simulink model "RLC_with_HBrdige_forward_circuit"  (R2022a)
settings: Solver=FixedStepAuto  StartTime=0.0  StopTime=.004  FixedStep=1e-6  RelTol=1e-3
values from neighbouring files (symbols this model uses):
  amplitude = 1200/pi    (= 381.971863421)    [RLC_Square_Wave_Driver.m]
  period = loc_nada(3) - loc_nada(1)    [Phase_shifting.m]    (also in RLC_Square_Wave_Driver.m = 1/i)
  RunTime = .004    (= 0.004)    [All_injectors_LQG_bop_plasma_ss_model_code.m]    (also in All_injectors_LQG_bop_ss_model_code.m; All_injectors_LQG_continuous_time_code.m; All_injectors_LQG_plasma_7_15_24_code.m; All_injectors_LQG_plasma_ss_model_code.m)
libraries: spsSeriesRLCBranchLib x8, spsMosfetLib x4, spsVoltageMeasurementLib x4, spsDCVoltageSourceLib x3, spsFullBridgeMMCExternalDCLinksLib x2, spsOnDelayLib x2, spsPWMGeneratorMultilevelLib x2, spsCurrentMeasurementLib x2, simulink x1, spspowerguiLib x1
settings Model: Creator=ducks  LastModifiedBy=ducks
settings DataIOCC: ExternalInput=[t,V]

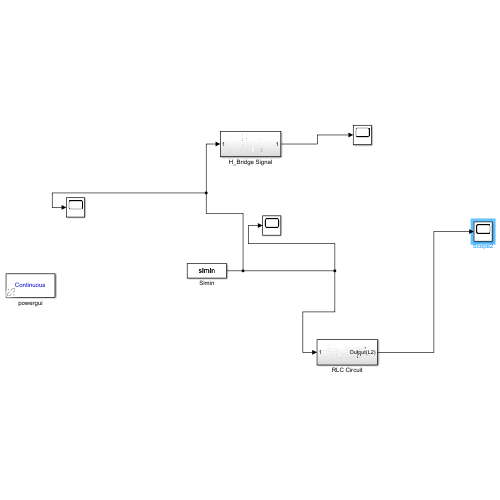
[thumbnail: Simulink's stored preview of the top-level diagram]
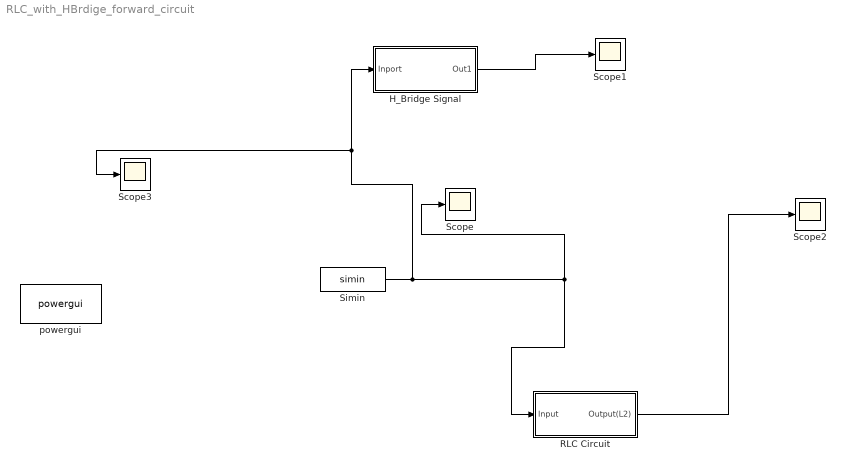
== system RLC_with_HBrdige_forward_circuit ==
  H_Bridge Signal : Subsystem
  RLC Circuit : Subsystem
  Scope{,1..3} (4 alike) : Scope
  Simin : FromWorkspace  VariableName=simin
  powergui : spspowerguiLib/powergui  Priority=1  SimulationMode=Continuous  SampleTime=50e-6  frequency=60  Iterations=50  frequencyindice=0  Pbase=100e6  ErrMax=1e-4  UnitsV=kV  UnitsW=MW  buscounter=0  FunctionMessages=off  echomessages=off  EnableUseOfTLC=off  CurrentSourceSwitches=off  DisableSnubberDevices=off  DisableRonSwitches=off  DisableVfSwitches=off  DisplayEquations=off  AutomaticDiscreteSolvers=off  SolverType=Tustin/Backward Euler (TBE)  Interpol=off  ExternalGateDelay=off  methode=off  Ts=100  x0status=blocks  SPID=on  SwTol=0  HookPort=off  NonlinearTolerance=1e-4  nMaxIteration=100  ContinueOnMaxIteration=off  RestoreLinks=warning  ResistiveCurrentMeasurement=off  Frange=[0:2:500]  Ylog=off  Xlog=on  ShowGrid=off  save=off  variable=ZData  structure=0  ZoomFFT=off  StartTime=0.0  cycles=1  DisplayStyle=1  fundamental=60  FreqAxis=off  MaxFrequency=1000  frequencyindicesteady=1  RmsSteady=1  display=off
  wires:
  Simin/1 -> Scope3/1, H_Bridge Signal/1(Inport), Scope/1, RLC Circuit/1(Input)
  H_Bridge Signal/1(Out1) -> Scope1/1
  RLC Circuit/1(Output(L2)) -> Scope2/1

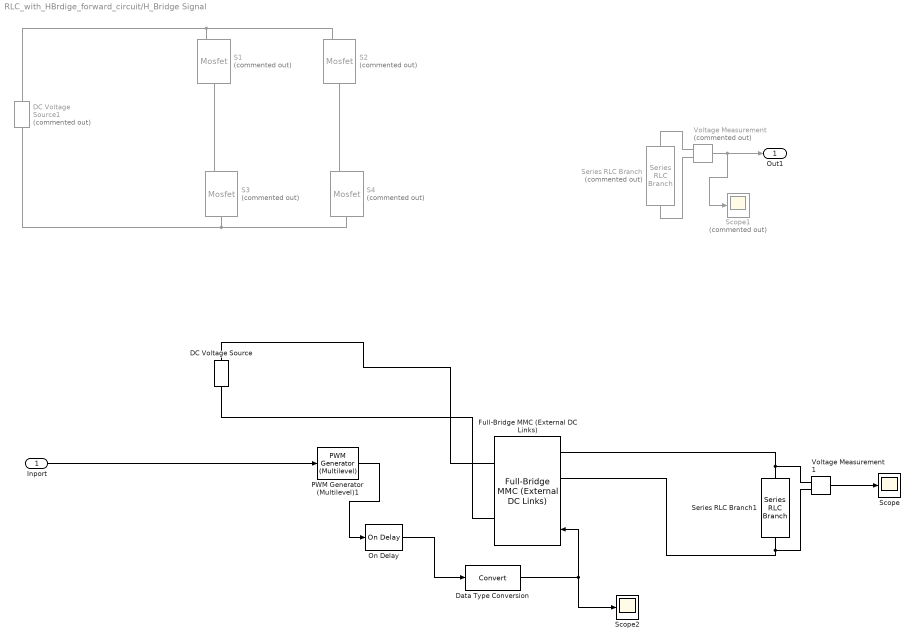
== system RLC_with_HBrdige_forward_circuit/H_Bridge Signal ==
  Inport : Inport
  DC Voltage Source : spsDCVoltageSourceLib/DC Voltage Source  Amplitude=600  Measurements=None
  DC Voltage Source1 : spsDCVoltageSourceLib/DC Voltage Source  Commented=on  Amplitude=600  Measurements=None
  Data Type Conversion : DataTypeConversion  SaturateOnIntegerOverflow=off  RndMeth=Floor
  Full-Bridge MMC (External DC Links) : spsFullBridgeMMCExternalDCLinksLib/Full-Bridge MMC (External DC Links)  ModelType=Switching devices  n=1  Ron=1e-3  Rs=1e6  Cs=inf  Ron_Diode=1e-3  Rs_Diode=1e6  Cs_Diode=inf  Vf_Diode=1e-3  Rs_CurrentSource=inf  Ts=10e-6
      settings: SourceProductBaseCode=PS
  On Delay : spsOnDelayLib/On Delay  DelayType=On delay  delay=.05*period  ic=0  Ts=0
      settings: SourceProductBaseCode=PS
  PWM Generator (Multilevel)1 : spsPWMGeneratorMultilevelLib/PWM Generator (Multilevel)  BridgeType=Full-bridge  NumberOfBridges=1  Fc=1e3  Ts=0  ShowCarriersOutport=off
      settings: SourceProductBaseCode=PS
  S{1..4} (4 alike) : spsMosfetLib/Mosfet  Commented=on  Ron=0.1  Lon=0  Rd=0.01  Vfd=0  IC=0  Rs=1e5  Cs=inf  Measurements=off
  Scope : Scope
  Scope1 : Scope  Commented=on
  Scope2 : Scope
  Series RLC Branch : spsSeriesRLCBranchLib/Series RLC Branch  Commented=on  LConnTagsString=__new0  RConnTagsString=__new0  BranchType=R  Resistance=1  Inductance=1e-3  SetiL0=off  InitialCurrent=0  Capacitance=1e-6  Setx0=off  InitialVoltage=0  Measurements=None
  Series RLC Branch1 : spsSeriesRLCBranchLib/Series RLC Branch  LConnTagsString=__new0  RConnTagsString=__new0  BranchType=R  Resistance=1  Inductance=1e-3  SetiL0=off  InitialCurrent=0  Capacitance=1e-6  Setx0=off  InitialVoltage=0  Measurements=None
  Voltage Measurement : spsVoltageMeasurementLib/Voltage Measurement  Commented=on  PhasorSimulation=off  OutputType=Complex  PSBequivalent=0
  Voltage Measurement1 : spsVoltageMeasurementLib/Voltage Measurement  PhasorSimulation=off  OutputType=Complex  PSBequivalent=0
  Out1 : Outport
  wires:
  Voltage Measurement/1 -> Scope1/1, Out1/1
  On Delay/1 -> Data Type Conversion/1
  PWM Generator (Multilevel)1/1 -> On Delay/1
  Inport/1 -> PWM Generator (Multilevel)1/1
  Data Type Conversion/1 -> Full-Bridge MMC (External DC Links)/1, Scope2/1
  Voltage Measurement1/1 -> Scope/1
  connections:
  Voltage Measurement/LConn1 -- Series RLC Branch/LConn1
  Voltage Measurement/LConn2 -- Series RLC Branch/RConn1
  S1/LConn1 -- S2/LConn1 -- DC Voltage Source1/LConn1
  S1/RConn1 -- S3/LConn1
  S3/RConn1 -- DC Voltage Source1/RConn1 -- S4/RConn1
  S4/LConn1 -- S2/RConn1
  Full-Bridge MMC (External DC Links)/LConn1 -- Voltage Measurement1/LConn2 -- Series RLC Branch1/RConn1
  Full-Bridge MMC (External DC Links)/RConn2 -- DC Voltage Source/LConn1
  Full-Bridge MMC (External DC Links)/LConn2 -- Voltage Measurement1/LConn1 -- Series RLC Branch1/LConn1
  Full-Bridge MMC (External DC Links)/RConn1 -- DC Voltage Source/RConn1

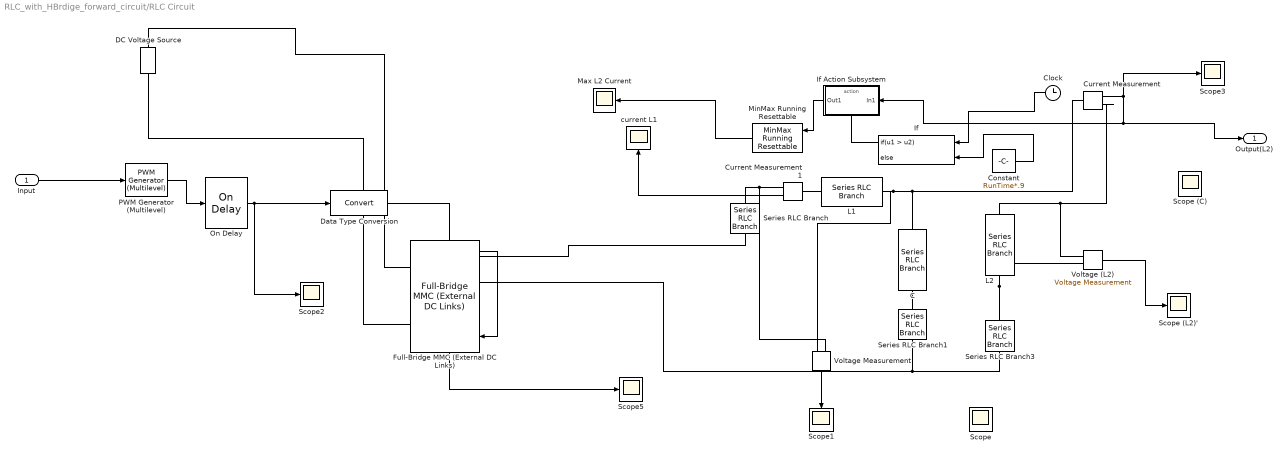
== system RLC_with_HBrdige_forward_circuit/RLC Circuit ==
  Input : Inport
  C : spsSeriesRLCBranchLib/Series RLC Branch  LConnTagsString=__new0  RConnTagsString=__new0  BranchType=C  Resistance=1  Inductance=1e-3  SetiL0=off  InitialCurrent=0  Capacitance=96e-6  Setx0=off  InitialVoltage=0  Measurements=None
  Clock : Clock
  Constant : Constant  Value=RunTime*.9
  Current Measurement : spsCurrentMeasurementLib/Current Measurement  PhasorSimulation=off  OutputType=Complex  PSBequivalent=0
  Current Measurement1 : spsCurrentMeasurementLib/Current Measurement  PhasorSimulation=off  OutputType=Complex  PSBequivalent=0
  DC Voltage Source : spsDCVoltageSourceLib/DC Voltage Source  Amplitude=amplitude  Measurements=None
  Data Type Conversion : DataTypeConversion  SaturateOnIntegerOverflow=off  RndMeth=Floor
  Full-Bridge MMC (External DC Links) : spsFullBridgeMMCExternalDCLinksLib/Full-Bridge MMC (External DC Links)  ModelType=Switching devices  n=1  Ron=1e-3  Rs=1e6  Cs=inf  Ron_Diode=1e-3  Rs_Diode=1e6  Cs_Diode=inf  Vf_Diode=1e-3  Rs_CurrentSource=inf  Ts=1e-6
      settings: SourceProductBaseCode=PS
  If : If  NumInputs=2  IfExpression=u1 > u2
  If Action Subsystem : Subsystem  TreatAsAtomicUnit=on
  L1 : spsSeriesRLCBranchLib/Series RLC Branch  LConnTagsString=__new0  RConnTagsString=__new0  BranchType=L  Resistance=1  Inductance=1.4e-6  SetiL0=off  InitialCurrent=0  Capacitance=0  Setx0=off  InitialVoltage=0  Measurements=None
  L2 : spsSeriesRLCBranchLib/Series RLC Branch  LConnTagsString=__new0  RConnTagsString=__new0  BranchType=L  Resistance=1  Inductance=1.5e-6  SetiL0=off  InitialCurrent=0  Capacitance=1e-6  Setx0=off  InitialVoltage=0  Measurements=None
  Max L2 Current : Scope
  MinMax Running Resettable : simulink/Math Operations/MinMax Running Resettable  Function=max  vinit=0.0
  On Delay : spsOnDelayLib/On Delay  DelayType=On delay  delay=.07*period  ic=0  Ts=0
      settings: SourceProductBaseCode=PS
  PWM Generator (Multilevel) : spsPWMGeneratorMultilevelLib/PWM Generator (Multilevel)  BridgeType=Full-bridge  NumberOfBridges=1  Fc=1e3  Ts=0  ShowCarriersOutport=off
      settings: SourceProductBaseCode=PS
  Scope{,1..3,5} (5 alike) : Scope
  Scope (C) : Scope
  Scope (L2)' : Scope
  Series RLC Branch : spsSeriesRLCBranchLib/Series RLC Branch  LConnTagsString=__new0  RConnTagsString=__new0  BranchType=R  Resistance=.0025  Inductance=1e-3  SetiL0=off  InitialCurrent=0  Capacitance=1e-6  Setx0=off  InitialVoltage=0  Measurements=None
  Series RLC Branch1 : spsSeriesRLCBranchLib/Series RLC Branch  LConnTagsString=__new0  RConnTagsString=__new0  BranchType=R  Resistance=.005  Inductance=1e-3  SetiL0=off  InitialCurrent=0  Capacitance=1e-6  Setx0=off  InitialVoltage=0  Measurements=None
  Series RLC Branch3 : spsSeriesRLCBranchLib/Series RLC Branch  LConnTagsString=__new0  RConnTagsString=__new0  BranchType=R  Resistance=.005  Inductance=1e-3  SetiL0=off  InitialCurrent=0  Capacitance=1e-6  Setx0=off  InitialVoltage=0  Measurements=None
  Voltage (L2) : spsVoltageMeasurementLib/Voltage Measurement  PhasorSimulation=off  OutputType=Complex  PSBequivalent=0
  Voltage Measurement : spsVoltageMeasurementLib/Voltage Measurement  PhasorSimulation=off  OutputType=Complex  PSBequivalent=0
  current L1 : Scope
  Output(L2) : Outport
  wires:
  Voltage Measurement/1 -> Scope1/1
  Voltage (L2)/1 -> Scope (L2)'/1
  Current Measurement1/1 -> current L1/1
  MinMax Running Resettable/1 -> Max L2 Current/1
  Clock/1 -> If/1
  Constant/1 -> If/2
  If/1 -> If Action Subsystem/Action
  If Action Subsystem/1(Out1) -> MinMax Running Resettable/1
  On Delay/1 -> Scope2/1, Data Type Conversion/1
  Data Type Conversion/1 -> Scope5/1, Full-Bridge MMC (External DC Links)/1
  PWM Generator (Multilevel)/1 -> On Delay/1
  Input/1 -> PWM Generator (Multilevel)/1
  Current Measurement/1 -> Output(L2)/1, If Action Subsystem/1(In1), Scope3/1
  connections:
  Current Measurement1/RConn1 -- Series RLC Branch/LConn1 -- Voltage Measurement/LConn1
  L2/RConn1 -- Voltage (L2)/LConn2 -- Series RLC Branch3/LConn1
  L1/LConn1 -- Current Measurement1/LConn1
  Voltage Measurement/LConn2 -- L1/RConn1 -- Current Measurement/LConn1 -- C/LConn1
  Current Measurement/RConn1 -- L2/LConn1 -- Voltage (L2)/LConn1
  Full-Bridge MMC (External DC Links)/LConn1 -- Series RLC Branch1/RConn1 -- Series RLC Branch3/RConn1
  Full-Bridge MMC (External DC Links)/RConn1 -- DC Voltage Source/RConn1
  Full-Bridge MMC (External DC Links)/RConn2 -- DC Voltage Source/LConn1
  Full-Bridge MMC (External DC Links)/LConn2 -- Series RLC Branch/RConn1
  Series RLC Branch1/LConn1 -- C/RConn1

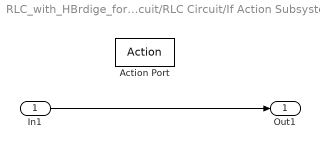
== system RLC_with_HBrdige_forward_circuit/RLC Circuit/If Action Subsystem ==
  In1 : Inport
  Action Port : ActionPort  ActionPortLabel=if(u1 > u2)
  Out1 : Outport
  wires:
  In1/1 -> Out1/1
